simulink model "MemCross3X5"  (R2018a)
settings: Solver=VariableStepAuto  StartTime=0.0  StopTime=10.0  RelTol=1e-3
libraries: components x9, fl_lib x8, nesl_utility x1
settings Model: Creator=dsentc  LastModifiedBy=dsentc

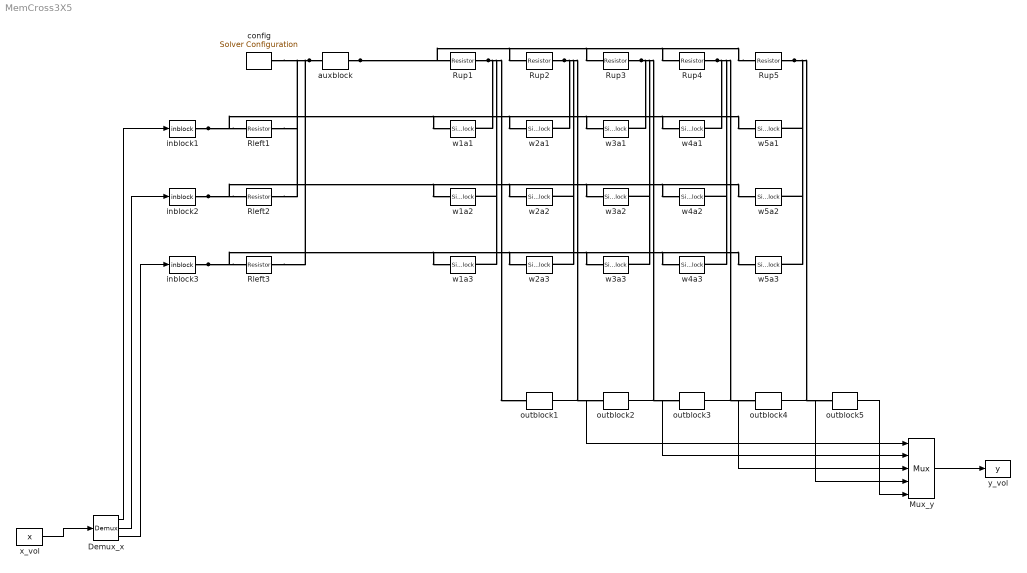
== system MemCross3X5 ==
  Demux_x : Demux  Outputs=3
  Mux_y : Mux  Inputs=5
  Rleft1 : fl_lib/Electrical/Electrical Elements/Resistor  R=2 Ohm  i_specify=off  i_priority=None  i=0 A  i_nominal_specify=off  i_nominal_unit=A  i_nominal_value=1  v_specify=off  v_priority=None  v=0 V  v_nominal_specify=off  v_nominal_unit=V  v_nominal_value=1
  Rleft2 : fl_lib/Electrical/Electrical Elements/Resistor  R=2 Ohm  i_specify=off  i_priority=None  i=0 A  i_nominal_specify=off  i_nominal_unit=A  i_nominal_value=1  v_specify=off  v_priority=None  v=0 V  v_nominal_specify=off  v_nominal_unit=V  v_nominal_value=1
  Rleft3 : fl_lib/Electrical/Electrical Elements/Resistor  R=2 Ohm  i_specify=off  i_priority=None  i=0 A  i_nominal_specify=off  i_nominal_unit=A  i_nominal_value=1  v_specify=off  v_priority=None  v=0 V  v_nominal_specify=off  v_nominal_unit=V  v_nominal_value=1
  Rup{1..5} (5 alike) : fl_lib/Electrical/Electrical Elements/Resistor  R=2 Ohm  i_specify=off  i_priority=None  i=0 A  i_nominal_specify=off  i_nominal_unit=A  i_nominal_value=1  v_specify=off  v_priority=None  v=0 V  v_nominal_specify=off  v_nominal_unit=V  v_nominal_value=1
  auxblock : components/auxblock
  config : nesl_utility/Solver Configuration  PhysicalDomain=network_engine_domain  SubClassName=solver  LeftPortType=input  RightPortType=generic  Tones=[]  Harmonics=[]  SimulateNoise=off  Profile=off  UseLocalSampling=off  EnableSwitchedLinearOptims=on  FrequencyDomain=off  UseCCode=off  RelTol=0.001  AbsTol=1e-06  MinStep=1e-09  ToWorkspace=off  RevertToSquareIcSolve=off  NumHomotopyIterations=100  PhasorMode=off  PhasorModeNumHarmonics=1  DoDC=off  ResidualTolerance=1e-09  UseLocalSolver=off  LocalSolverChoice=NE_BACKWARD_EULER_ADVANCER  LocalSolverSampleTime=0.001  DoFixedCost=off  MaxNonlinIter=3  MaxModeIter=2  LinearAlgebra=Sparse  EquationFormulation=NE_TIME_EF  DelaysMemoryBudget=1024  AutomaticFiltering=on  FilteringTimeConstant=0.001
  inblock1 : components/inblock
  inblock2 : components/inblock
  inblock3 : components/inblock
  outblock{1..5} (5 alike) : components/outblock
  w1a1 : SimscapeComponentBlock  SourceFile=Memristor_ideal.Memristor_ideal  ComponentPath=Memristor_ideal.Memristor_ideal  ComponentVariants=Memristor_ideal.Memristor_ideal  ComponentVariantNames=Memristor_ideal  ClassName=Memristor_ideal  SchemaVersion=1  G1=0.9999 S  G0=0.0001 S  v_off=1 V  v_on=-1 V  w0=0  c1=1 V  c2=9.999e-6 s*V  w_specify=off  w_priority=None  w=0  w_nominal_specify=off  w_nominal_unit=1  w_nominal_value=1  i_specify=off  i_priority=None  i=0 A  i_nominal_specify=off  i_nominal_unit=A  i_nominal_value=1  v_specify=off  v_priority=None  v=0 V  v_nominal_specify=off  v_nominal_unit=V  v_nominal_value=1  power_dissipated_specify=off  power_dissipated_priority=None  power_dissipated=0 W  power_dissipated_nominal_specify=off  power_dissipated_nominal_unit=W  power_dissipated_nominal_value=1
      settings: CopyFcn=simscape.engine.sli.internal.componentblockcallback(gcbh,'COPY')  PreCopyFcn=simscape.engine.sli.internal.componentblockcallback(gcbh,'PRECOPY')  PreDeleteFcn=simscape.engine.sli.internal.componentblockcallback(gcbh,'PREDELETE')
      mask Type: memristor_ideal
  w1a2 : SimscapeComponentBlock  SourceFile=Memristor_ideal.Memristor_ideal  ComponentPath=Memristor_ideal.Memristor_ideal  ComponentVariants=Memristor_ideal.Memristor_ideal  ComponentVariantNames=Memristor_ideal  ClassName=Memristor_ideal  SchemaVersion=1  G1=0.9999 S  G0=0.0001 S  v_off=1 V  v_on=-1 V  w0=0  c1=1 V  c2=9.999e-6 s*V  w_specify=off  w_priority=None  w=0  w_nominal_specify=off  w_nominal_unit=1  w_nominal_value=1  i_specify=off  i_priority=None  i=0 A  i_nominal_specify=off  i_nominal_unit=A  i_nominal_value=1  v_specify=off  v_priority=None  v=0 V  v_nominal_specify=off  v_nominal_unit=V  v_nominal_value=1  power_dissipated_specify=off  power_dissipated_priority=None  power_dissipated=0 W  power_dissipated_nominal_specify=off  power_dissipated_nominal_unit=W  power_dissipated_nominal_value=1
      settings: CopyFcn=simscape.engine.sli.internal.componentblockcallback(gcbh,'COPY')  PreCopyFcn=simscape.engine.sli.internal.componentblockcallback(gcbh,'PRECOPY')  PreDeleteFcn=simscape.engine.sli.internal.componentblockcallback(gcbh,'PREDELETE')
      mask Type: memristor_ideal
  w1a3 : SimscapeComponentBlock  SourceFile=Memristor_ideal.Memristor_ideal  ComponentPath=Memristor_ideal.Memristor_ideal  ComponentVariants=Memristor_ideal.Memristor_ideal  ComponentVariantNames=Memristor_ideal  ClassName=Memristor_ideal  SchemaVersion=1  G1=0.9999 S  G0=0.0001 S  v_off=1 V  v_on=-1 V  w0=0  c1=1 V  c2=9.999e-6 s*V  w_specify=off  w_priority=None  w=0  w_nominal_specify=off  w_nominal_unit=1  w_nominal_value=1  i_specify=off  i_priority=None  i=0 A  i_nominal_specify=off  i_nominal_unit=A  i_nominal_value=1  v_specify=off  v_priority=None  v=0 V  v_nominal_specify=off  v_nominal_unit=V  v_nominal_value=1  power_dissipated_specify=off  power_dissipated_priority=None  power_dissipated=0 W  power_dissipated_nominal_specify=off  power_dissipated_nominal_unit=W  power_dissipated_nominal_value=1
      settings: CopyFcn=simscape.engine.sli.internal.componentblockcallback(gcbh,'COPY')  PreCopyFcn=simscape.engine.sli.internal.componentblockcallback(gcbh,'PRECOPY')  PreDeleteFcn=simscape.engine.sli.internal.componentblockcallback(gcbh,'PREDELETE')
      mask Type: memristor_ideal
  w2a1 : SimscapeComponentBlock  SourceFile=Memristor_ideal.Memristor_ideal  ComponentPath=Memristor_ideal.Memristor_ideal  ComponentVariants=Memristor_ideal.Memristor_ideal  ComponentVariantNames=Memristor_ideal  ClassName=Memristor_ideal  SchemaVersion=1  G1=0.9999 S  G0=0.0001 S  v_off=1 V  v_on=-1 V  w0=0  c1=1 V  c2=9.999e-6 s*V  w_specify=off  w_priority=None  w=0  w_nominal_specify=off  w_nominal_unit=1  w_nominal_value=1  i_specify=off  i_priority=None  i=0 A  i_nominal_specify=off  i_nominal_unit=A  i_nominal_value=1  v_specify=off  v_priority=None  v=0 V  v_nominal_specify=off  v_nominal_unit=V  v_nominal_value=1  power_dissipated_specify=off  power_dissipated_priority=None  power_dissipated=0 W  power_dissipated_nominal_specify=off  power_dissipated_nominal_unit=W  power_dissipated_nominal_value=1
      settings: CopyFcn=simscape.engine.sli.internal.componentblockcallback(gcbh,'COPY')  PreCopyFcn=simscape.engine.sli.internal.componentblockcallback(gcbh,'PRECOPY')  PreDeleteFcn=simscape.engine.sli.internal.componentblockcallback(gcbh,'PREDELETE')
      mask Type: memristor_ideal
  w2a2 : SimscapeComponentBlock  SourceFile=Memristor_ideal.Memristor_ideal  ComponentPath=Memristor_ideal.Memristor_ideal  ComponentVariants=Memristor_ideal.Memristor_ideal  ComponentVariantNames=Memristor_ideal  ClassName=Memristor_ideal  SchemaVersion=1  G1=0.9999 S  G0=0.0001 S  v_off=1 V  v_on=-1 V  w0=0  c1=1 V  c2=9.999e-6 s*V  w_specify=off  w_priority=None  w=0  w_nominal_specify=off  w_nominal_unit=1  w_nominal_value=1  i_specify=off  i_priority=None  i=0 A  i_nominal_specify=off  i_nominal_unit=A  i_nominal_value=1  v_specify=off  v_priority=None  v=0 V  v_nominal_specify=off  v_nominal_unit=V  v_nominal_value=1  power_dissipated_specify=off  power_dissipated_priority=None  power_dissipated=0 W  power_dissipated_nominal_specify=off  power_dissipated_nominal_unit=W  power_dissipated_nominal_value=1
      settings: CopyFcn=simscape.engine.sli.internal.componentblockcallback(gcbh,'COPY')  PreCopyFcn=simscape.engine.sli.internal.componentblockcallback(gcbh,'PRECOPY')  PreDeleteFcn=simscape.engine.sli.internal.componentblockcallback(gcbh,'PREDELETE')
      mask Type: memristor_ideal
  w2a3 : SimscapeComponentBlock  SourceFile=Memristor_ideal.Memristor_ideal  ComponentPath=Memristor_ideal.Memristor_ideal  ComponentVariants=Memristor_ideal.Memristor_ideal  ComponentVariantNames=Memristor_ideal  ClassName=Memristor_ideal  SchemaVersion=1  G1=0.9999 S  G0=0.0001 S  v_off=1 V  v_on=-1 V  w0=0  c1=1 V  c2=9.999e-6 s*V  w_specify=off  w_priority=None  w=0  w_nominal_specify=off  w_nominal_unit=1  w_nominal_value=1  i_specify=off  i_priority=None  i=0 A  i_nominal_specify=off  i_nominal_unit=A  i_nominal_value=1  v_specify=off  v_priority=None  v=0 V  v_nominal_specify=off  v_nominal_unit=V  v_nominal_value=1  power_dissipated_specify=off  power_dissipated_priority=None  power_dissipated=0 W  power_dissipated_nominal_specify=off  power_dissipated_nominal_unit=W  power_dissipated_nominal_value=1
      settings: CopyFcn=simscape.engine.sli.internal.componentblockcallback(gcbh,'COPY')  PreCopyFcn=simscape.engine.sli.internal.componentblockcallback(gcbh,'PRECOPY')  PreDeleteFcn=simscape.engine.sli.internal.componentblockcallback(gcbh,'PREDELETE')
      mask Type: memristor_ideal
  w3a1 : SimscapeComponentBlock  SourceFile=Memristor_ideal.Memristor_ideal  ComponentPath=Memristor_ideal.Memristor_ideal  ComponentVariants=Memristor_ideal.Memristor_ideal  ComponentVariantNames=Memristor_ideal  ClassName=Memristor_ideal  SchemaVersion=1  G1=0.9999 S  G0=0.0001 S  v_off=1 V  v_on=-1 V  w0=0  c1=1 V  c2=9.999e-6 s*V  w_specify=off  w_priority=None  w=0  w_nominal_specify=off  w_nominal_unit=1  w_nominal_value=1  i_specify=off  i_priority=None  i=0 A  i_nominal_specify=off  i_nominal_unit=A  i_nominal_value=1  v_specify=off  v_priority=None  v=0 V  v_nominal_specify=off  v_nominal_unit=V  v_nominal_value=1  power_dissipated_specify=off  power_dissipated_priority=None  power_dissipated=0 W  power_dissipated_nominal_specify=off  power_dissipated_nominal_unit=W  power_dissipated_nominal_value=1
      settings: CopyFcn=simscape.engine.sli.internal.componentblockcallback(gcbh,'COPY')  PreCopyFcn=simscape.engine.sli.internal.componentblockcallback(gcbh,'PRECOPY')  PreDeleteFcn=simscape.engine.sli.internal.componentblockcallback(gcbh,'PREDELETE')
      mask Type: memristor_ideal
  w3a2 : SimscapeComponentBlock  SourceFile=Memristor_ideal.Memristor_ideal  ComponentPath=Memristor_ideal.Memristor_ideal  ComponentVariants=Memristor_ideal.Memristor_ideal  ComponentVariantNames=Memristor_ideal  ClassName=Memristor_ideal  SchemaVersion=1  G1=0.9999 S  G0=0.0001 S  v_off=1 V  v_on=-1 V  w0=0  c1=1 V  c2=9.999e-6 s*V  w_specify=off  w_priority=None  w=0  w_nominal_specify=off  w_nominal_unit=1  w_nominal_value=1  i_specify=off  i_priority=None  i=0 A  i_nominal_specify=off  i_nominal_unit=A  i_nominal_value=1  v_specify=off  v_priority=None  v=0 V  v_nominal_specify=off  v_nominal_unit=V  v_nominal_value=1  power_dissipated_specify=off  power_dissipated_priority=None  power_dissipated=0 W  power_dissipated_nominal_specify=off  power_dissipated_nominal_unit=W  power_dissipated_nominal_value=1
      settings: CopyFcn=simscape.engine.sli.internal.componentblockcallback(gcbh,'COPY')  PreCopyFcn=simscape.engine.sli.internal.componentblockcallback(gcbh,'PRECOPY')  PreDeleteFcn=simscape.engine.sli.internal.componentblockcallback(gcbh,'PREDELETE')
      mask Type: memristor_ideal
  w3a3 : SimscapeComponentBlock  SourceFile=Memristor_ideal.Memristor_ideal  ComponentPath=Memristor_ideal.Memristor_ideal  ComponentVariants=Memristor_ideal.Memristor_ideal  ComponentVariantNames=Memristor_ideal  ClassName=Memristor_ideal  SchemaVersion=1  G1=0.9999 S  G0=0.0001 S  v_off=1 V  v_on=-1 V  w0=0  c1=1 V  c2=9.999e-6 s*V  w_specify=off  w_priority=None  w=0  w_nominal_specify=off  w_nominal_unit=1  w_nominal_value=1  i_specify=off  i_priority=None  i=0 A  i_nominal_specify=off  i_nominal_unit=A  i_nominal_value=1  v_specify=off  v_priority=None  v=0 V  v_nominal_specify=off  v_nominal_unit=V  v_nominal_value=1  power_dissipated_specify=off  power_dissipated_priority=None  power_dissipated=0 W  power_dissipated_nominal_specify=off  power_dissipated_nominal_unit=W  power_dissipated_nominal_value=1
      settings: CopyFcn=simscape.engine.sli.internal.componentblockcallback(gcbh,'COPY')  PreCopyFcn=simscape.engine.sli.internal.componentblockcallback(gcbh,'PRECOPY')  PreDeleteFcn=simscape.engine.sli.internal.componentblockcallback(gcbh,'PREDELETE')
      mask Type: memristor_ideal
  w4a1 : SimscapeComponentBlock  SourceFile=Memristor_ideal.Memristor_ideal  ComponentPath=Memristor_ideal.Memristor_ideal  ComponentVariants=Memristor_ideal.Memristor_ideal  ComponentVariantNames=Memristor_ideal  ClassName=Memristor_ideal  SchemaVersion=1  G1=0.9999 S  G0=0.0001 S  v_off=1 V  v_on=-1 V  w0=0  c1=1 V  c2=9.999e-6 s*V  w_specify=off  w_priority=None  w=0  w_nominal_specify=off  w_nominal_unit=1  w_nominal_value=1  i_specify=off  i_priority=None  i=0 A  i_nominal_specify=off  i_nominal_unit=A  i_nominal_value=1  v_specify=off  v_priority=None  v=0 V  v_nominal_specify=off  v_nominal_unit=V  v_nominal_value=1  power_dissipated_specify=off  power_dissipated_priority=None  power_dissipated=0 W  power_dissipated_nominal_specify=off  power_dissipated_nominal_unit=W  power_dissipated_nominal_value=1
      settings: CopyFcn=simscape.engine.sli.internal.componentblockcallback(gcbh,'COPY')  PreCopyFcn=simscape.engine.sli.internal.componentblockcallback(gcbh,'PRECOPY')  PreDeleteFcn=simscape.engine.sli.internal.componentblockcallback(gcbh,'PREDELETE')
      mask Type: memristor_ideal
  w4a2 : SimscapeComponentBlock  SourceFile=Memristor_ideal.Memristor_ideal  ComponentPath=Memristor_ideal.Memristor_ideal  ComponentVariants=Memristor_ideal.Memristor_ideal  ComponentVariantNames=Memristor_ideal  ClassName=Memristor_ideal  SchemaVersion=1  G1=0.9999 S  G0=0.0001 S  v_off=1 V  v_on=-1 V  w0=0  c1=1 V  c2=9.999e-6 s*V  w_specify=off  w_priority=None  w=0  w_nominal_specify=off  w_nominal_unit=1  w_nominal_value=1  i_specify=off  i_priority=None  i=0 A  i_nominal_specify=off  i_nominal_unit=A  i_nominal_value=1  v_specify=off  v_priority=None  v=0 V  v_nominal_specify=off  v_nominal_unit=V  v_nominal_value=1  power_dissipated_specify=off  power_dissipated_priority=None  power_dissipated=0 W  power_dissipated_nominal_specify=off  power_dissipated_nominal_unit=W  power_dissipated_nominal_value=1
      settings: CopyFcn=simscape.engine.sli.internal.componentblockcallback(gcbh,'COPY')  PreCopyFcn=simscape.engine.sli.internal.componentblockcallback(gcbh,'PRECOPY')  PreDeleteFcn=simscape.engine.sli.internal.componentblockcallback(gcbh,'PREDELETE')
      mask Type: memristor_ideal
  w4a3 : SimscapeComponentBlock  SourceFile=Memristor_ideal.Memristor_ideal  ComponentPath=Memristor_ideal.Memristor_ideal  ComponentVariants=Memristor_ideal.Memristor_ideal  ComponentVariantNames=Memristor_ideal  ClassName=Memristor_ideal  SchemaVersion=1  G1=0.9999 S  G0=0.0001 S  v_off=1 V  v_on=-1 V  w0=0  c1=1 V  c2=9.999e-6 s*V  w_specify=off  w_priority=None  w=0  w_nominal_specify=off  w_nominal_unit=1  w_nominal_value=1  i_specify=off  i_priority=None  i=0 A  i_nominal_specify=off  i_nominal_unit=A  i_nominal_value=1  v_specify=off  v_priority=None  v=0 V  v_nominal_specify=off  v_nominal_unit=V  v_nominal_value=1  power_dissipated_specify=off  power_dissipated_priority=None  power_dissipated=0 W  power_dissipated_nominal_specify=off  power_dissipated_nominal_unit=W  power_dissipated_nominal_value=1
      settings: CopyFcn=simscape.engine.sli.internal.componentblockcallback(gcbh,'COPY')  PreCopyFcn=simscape.engine.sli.internal.componentblockcallback(gcbh,'PRECOPY')  PreDeleteFcn=simscape.engine.sli.internal.componentblockcallback(gcbh,'PREDELETE')
      mask Type: memristor_ideal
  w5a1 : SimscapeComponentBlock  SourceFile=Memristor_ideal.Memristor_ideal  ComponentPath=Memristor_ideal.Memristor_ideal  ComponentVariants=Memristor_ideal.Memristor_ideal  ComponentVariantNames=Memristor_ideal  ClassName=Memristor_ideal  SchemaVersion=1  G1=0.9999 S  G0=0.0001 S  v_off=1 V  v_on=-1 V  w0=0  c1=1 V  c2=9.999e-6 s*V  w_specify=off  w_priority=None  w=0  w_nominal_specify=off  w_nominal_unit=1  w_nominal_value=1  i_specify=off  i_priority=None  i=0 A  i_nominal_specify=off  i_nominal_unit=A  i_nominal_value=1  v_specify=off  v_priority=None  v=0 V  v_nominal_specify=off  v_nominal_unit=V  v_nominal_value=1  power_dissipated_specify=off  power_dissipated_priority=None  power_dissipated=0 W  power_dissipated_nominal_specify=off  power_dissipated_nominal_unit=W  power_dissipated_nominal_value=1
      settings: CopyFcn=simscape.engine.sli.internal.componentblockcallback(gcbh,'COPY')  PreCopyFcn=simscape.engine.sli.internal.componentblockcallback(gcbh,'PRECOPY')  PreDeleteFcn=simscape.engine.sli.internal.componentblockcallback(gcbh,'PREDELETE')
      mask Type: memristor_ideal
  w5a2 : SimscapeComponentBlock  SourceFile=Memristor_ideal.Memristor_ideal  ComponentPath=Memristor_ideal.Memristor_ideal  ComponentVariants=Memristor_ideal.Memristor_ideal  ComponentVariantNames=Memristor_ideal  ClassName=Memristor_ideal  SchemaVersion=1  G1=0.9999 S  G0=0.0001 S  v_off=1 V  v_on=-1 V  w0=0  c1=1 V  c2=9.999e-6 s*V  w_specify=off  w_priority=None  w=0  w_nominal_specify=off  w_nominal_unit=1  w_nominal_value=1  i_specify=off  i_priority=None  i=0 A  i_nominal_specify=off  i_nominal_unit=A  i_nominal_value=1  v_specify=off  v_priority=None  v=0 V  v_nominal_specify=off  v_nominal_unit=V  v_nominal_value=1  power_dissipated_specify=off  power_dissipated_priority=None  power_dissipated=0 W  power_dissipated_nominal_specify=off  power_dissipated_nominal_unit=W  power_dissipated_nominal_value=1
      settings: CopyFcn=simscape.engine.sli.internal.componentblockcallback(gcbh,'COPY')  PreCopyFcn=simscape.engine.sli.internal.componentblockcallback(gcbh,'PRECOPY')  PreDeleteFcn=simscape.engine.sli.internal.componentblockcallback(gcbh,'PREDELETE')
      mask Type: memristor_ideal
  w5a3 : SimscapeComponentBlock  SourceFile=Memristor_ideal.Memristor_ideal  ComponentPath=Memristor_ideal.Memristor_ideal  ComponentVariants=Memristor_ideal.Memristor_ideal  ComponentVariantNames=Memristor_ideal  ClassName=Memristor_ideal  SchemaVersion=1  G1=0.9999 S  G0=0.0001 S  v_off=1 V  v_on=-1 V  w0=0  c1=1 V  c2=9.999e-6 s*V  w_specify=off  w_priority=None  w=0  w_nominal_specify=off  w_nominal_unit=1  w_nominal_value=1  i_specify=off  i_priority=None  i=0 A  i_nominal_specify=off  i_nominal_unit=A  i_nominal_value=1  v_specify=off  v_priority=None  v=0 V  v_nominal_specify=off  v_nominal_unit=V  v_nominal_value=1  power_dissipated_specify=off  power_dissipated_priority=None  power_dissipated=0 W  power_dissipated_nominal_specify=off  power_dissipated_nominal_unit=W  power_dissipated_nominal_value=1
      settings: CopyFcn=simscape.engine.sli.internal.componentblockcallback(gcbh,'COPY')  PreCopyFcn=simscape.engine.sli.internal.componentblockcallback(gcbh,'PRECOPY')  PreDeleteFcn=simscape.engine.sli.internal.componentblockcallback(gcbh,'PREDELETE')
      mask Type: memristor_ideal
  x_vol : FromWorkspace  VariableName=x  SampleTime=0
  y_vol : ToWorkspace  VariableName=y  SampleTime=-1
  wires:
  x_vol/1 -> Demux_x/1
  Demux_x/3 -> inblock3/1
  Demux_x/2 -> inblock2/1
  Demux_x/1 -> inblock1/1
  outblock5/1 -> Mux_y/5
  outblock4/1 -> Mux_y/4
  outblock3/1 -> Mux_y/3
  outblock2/1 -> Mux_y/2
  outblock1/1 -> Mux_y/1
  Mux_y/1 -> y_vol/1
  connections:
  Rleft3/LConn1 -- inblock3/RConn1 -- w1a3/LConn1 -- w2a3/LConn1 -- w3a3/LConn1 -- w4a3/LConn1 -- w5a3/LConn1
  Rleft3/RConn1 -- Rleft2/RConn1 -- Rleft1/RConn1 -- auxblock/LConn1 -- config/RConn1
  Rleft2/LConn1 -- inblock2/RConn1 -- w1a2/LConn1 -- w2a2/LConn1 -- w3a2/LConn1 -- w4a2/LConn1 -- w5a2/LConn1
  Rleft1/LConn1 -- inblock1/RConn1 -- w1a1/LConn1 -- w2a1/LConn1 -- w3a1/LConn1 -- w4a1/LConn1 -- w5a1/LConn1
  Rup5/LConn1 -- auxblock/RConn1 -- Rup4/LConn1 -- Rup3/LConn1 -- Rup2/LConn1 -- Rup1/LConn1
  w5a1/RConn1 -- Rup5/RConn1 -- w5a2/RConn1 -- w5a3/RConn1 -- outblock5/LConn1
  w4a1/RConn1 -- Rup4/RConn1 -- w4a2/RConn1 -- w4a3/RConn1 -- outblock4/LConn1
  w3a1/RConn1 -- Rup3/RConn1 -- w3a2/RConn1 -- w3a3/RConn1 -- outblock3/LConn1
  w2a1/RConn1 -- Rup2/RConn1 -- w2a2/RConn1 -- w2a3/RConn1 -- outblock2/LConn1
  w1a1/RConn1 -- Rup1/RConn1 -- w1a2/RConn1 -- w1a3/RConn1 -- outblock1/LConn1
